simulink model "gm_untitled"  (R2013a)
settings: Solver=ode45  StartTime=0.0  StopTime=20.0  RelTol=1e-3
settings Model: Creator=root  LastModifiedBy=root
settings OptimizationCC: BlockReduction=off  ConditionallyExecuteInputs=off

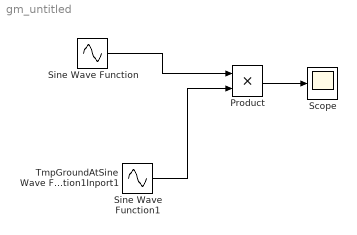
== system gm_untitled ==
  Product : Product
  Scope : Scope
  Sine Wave Function : Sin  Amplitude=6  Frequency=5  SampleTime=0
  Sine Wave Function1 : Sin  TimeSource=Use external signal  Amplitude=6  Frequency=200  Phase=2  SampleTime=0
  TmpGroundAtSine Wave Function1Inport1 : Ground  DisableCoverage=on
  wires:
  Product/1 -> Scope/1
  Sine Wave Function/1 -> Product/1
  Sine Wave Function1/1 -> Product/2
  TmpGroundAtSine Wave Function1Inport1/1 -> Sine Wave Function1/1
